simulink model "observer"  (R2022b)
settings: Solver=VariableStepAuto  StartTime=0.0  StopTime=200  RelTol=1e-3
undefined symbols (not defined in the file): A, B, C, L
settings Model: Creator=amoralesma  LastModifiedBy=amoralesma

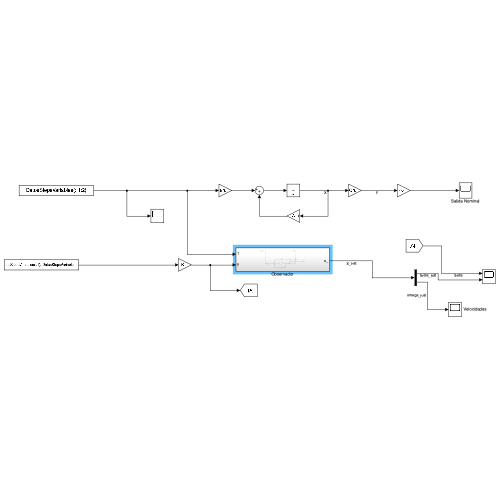
[thumbnail: Simulink's stored preview of the top-level diagram]
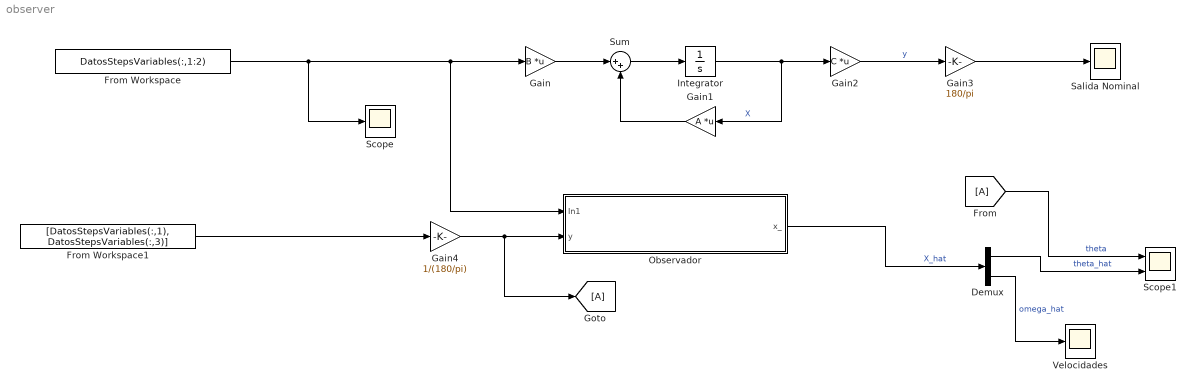
== system observer ==
  Demux : Demux  Outputs=2
  From : From
  From Workspace : FromWorkspace  VariableName=DatosStepsVariables(:,1:2)  SampleTime=2.5e-3
  From Workspace1 : FromWorkspace  VariableName=[DatosStepsVariables(:,1), DatosStepsVariables(:,3)]  SampleTime=2.5e-3
  Gain : Gain  Gain=B  Multiplication=Matrix(K*u)
  Gain1 : Gain  Gain=A  Multiplication=Matrix(K*u)
  Gain2 : Gain  Gain=C  Multiplication=Matrix(K*u)
  Gain3 : Gain  Gain=180/pi
  Gain4 : Gain  Gain=1/(180/pi)
  Goto : Goto
  Integrator : Integrator
  Observador : Subsystem
  Salida Nominal : Scope
  Scope : Scope
  Scope1 : Scope  NumInputPorts=2
  Sum : Sum  Inputs=|++
  Velocidades : Scope
  wires:
  Integrator/1 -> Gain1/1, Gain2/1  "X"
  Gain1/1 -> Sum/2
  Sum/1 -> Integrator/1
  Gain/1 -> Sum/1
  Gain2/1 -> Gain3/1  "y"
  From Workspace/1 -> Scope/1, Observador/1(In1), Gain/1
  Observador/1(x_) -> Demux/1  "X_hat"
  Gain3/1 -> Salida Nominal/1
  Gain4/1 -> Goto/1, Observador/2(y)
  Demux/1 -> Scope1/2  "theta_hat"
  From/1 -> Scope1/1  "theta"
  Demux/2 -> Velocidades/1  "omega_hat"
  From Workspace1/1 -> Gain4/1

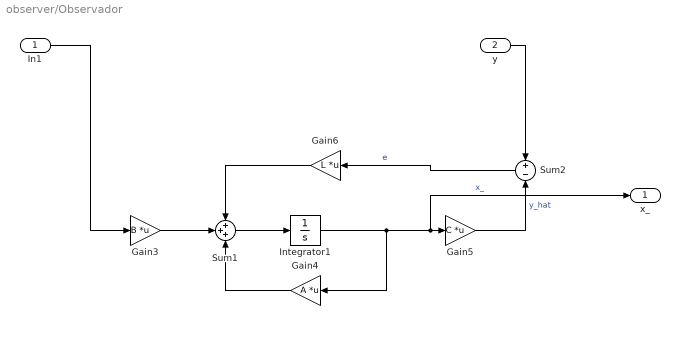
== system observer/Observador ==
  In1 : Inport
  y : Inport  Port=2
  Gain3 : Gain  Gain=B  Multiplication=Matrix(K*u)
  Gain4 : Gain  Gain=A  Multiplication=Matrix(K*u)
  Gain5 : Gain  Gain=C  Multiplication=Matrix(K*u)
  Gain6 : Gain  Gain=L  Multiplication=Matrix(K*u)
  Integrator1 : Integrator
  Sum1 : Sum  Inputs=+++
  Sum2 : Sum  Inputs=+|-
  x_ : Outport
  wires:
  In1/1 -> Gain3/1
  y/1 -> Sum2/1
  Gain5/1 -> Sum2/2  "y_hat"
  Sum1/1 -> Integrator1/1
  Gain3/1 -> Sum1/2
  Gain6/1 -> Sum1/1
  Integrator1/1 -> Gain4/1, x_/1, Gain5/1  "x_"
  Sum2/1 -> Gain6/1  "e"
  Gain4/1 -> Sum1/3
